simulink model "Ballschuss1"  (Simulink 7.1)
settings: Solver=ode45  StartTime=0.0  StopTime=4  RelTol=1e-3
settings Model: Creator=Meisel  LastModifiedBy=Meisel

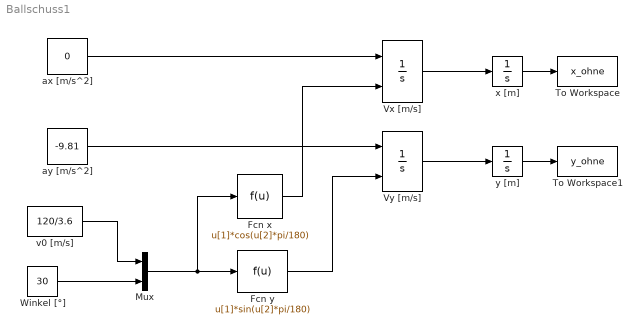
== system Ballschuss1 ==
  Fcn x : Fcn  Expr=u[1]*cos(u[2]*pi/180)
  Fcn y : Fcn  Expr=u[1]*sin(u[2]*pi/180)
  Mux : Mux  Inputs=2
  To Workspace : ToWorkspace  VariableName=x_ohne  SampleTime=-1  SaveFormat=Array
  To Workspace1 : ToWorkspace  VariableName=y_ohne  SampleTime=-1  SaveFormat=Array
  Vx [m/s] : Integrator  InitialConditionSource=external  InitialCondition=5
  Vy [m/s] : Integrator  InitialConditionSource=external  InitialCondition=5
  Winkel [°] : Constant  Value=30  OutDataType=sfix(16)  OutScaling=2^0
  ax [m/s^2] : Constant  Value=0  OutDataType=sfix(16)  OutScaling=2^0
  ay [m/s^2] : Constant  Value=-9.81  OutDataType=sfix(16)  OutScaling=2^0
  v0 [m/s] : Constant  Value=120/3.6  OutDataType=sfix(16)  OutScaling=2^0
  x [m] : Integrator
  y [m] : Integrator
  wires:
  ay [m/s^2]/1 -> Vy [m/s]/1
  Vy [m/s]/1 -> y [m]/1
  ax [m/s^2]/1 -> Vx [m/s]/1
  Vx [m/s]/1 -> x [m]/1
  Winkel [°]/1 -> Mux/2
  Fcn x/1 -> Vx [m/s]/2
  Fcn y/1 -> Vy [m/s]/2
  v0 [m/s]/1 -> Mux/1
  Mux/1 -> Fcn x/1, Fcn y/1
  x [m]/1 -> To Workspace/1
  y [m]/1 -> To Workspace1/1
